simulink model "simpleThermalModel_v2"  (R2022a)
settings: Solver=VariableStepAuto  StartTime=0.0  StopTime=36000  RelTol=1e-3
libraries: fl_lib x161, nesl_utility x51
(part 1 of 2)
settings Model: Creator=BrunoMattos  LastModifiedBy=BrunoMattos
settings OptimizationCC: ZeroExternalMemoryAtStartup=off  ZeroInternalMemoryAtStartup=off
settings RTWCC: TargetLang=C++
settings GRTTargetCC: TargetLangStandard=C++11 (ISO)  CodeInterfacePackaging=C++ class

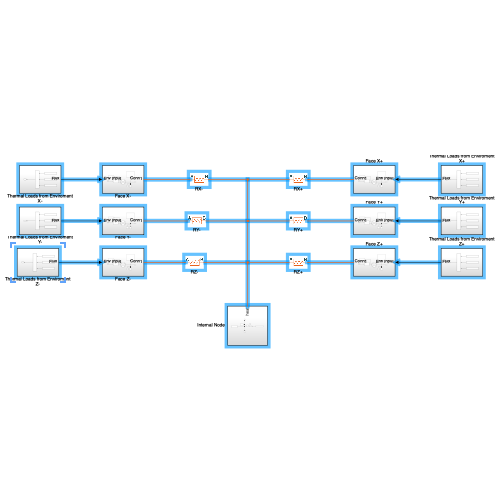
[thumbnail: Simulink's stored preview of the top-level diagram]
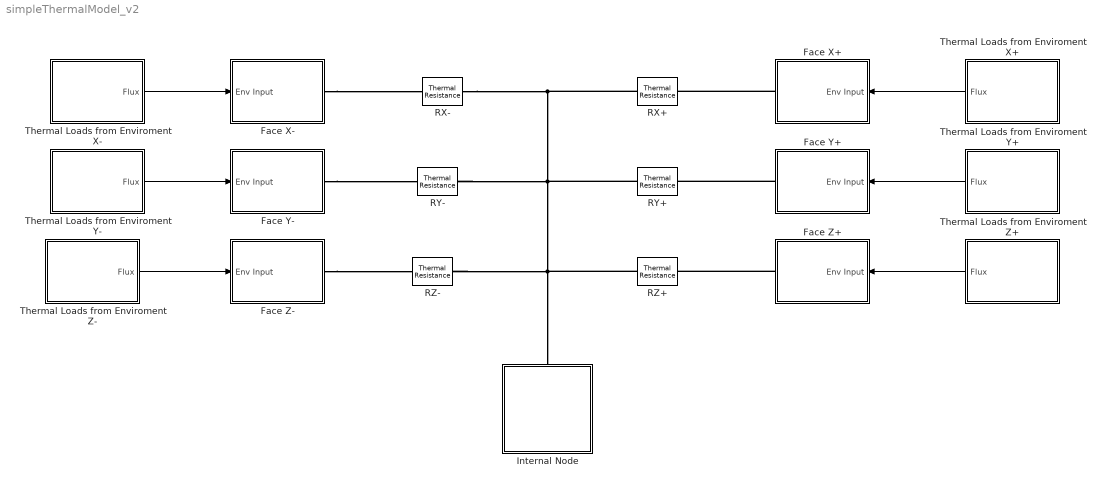
== system simpleThermalModel_v2 ==
  Face X+ : Subsystem
  Face X- : Subsystem
  Face Y+ : Subsystem
  Face Y- : Subsystem
  Face Z+ : Subsystem
  Face Z- : Subsystem
  Internal Node : Subsystem
  RX+ : fl_lib/Thermal/Thermal Elements/Thermal Resistance  resistance=0 K/W  T_specify=off  T_priority=None  T=0 K  T_nominal_specify=off  T_nominal_unit=K  T_nominal_value=1  Q_specify=off  Q_priority=None  Q=0 W  Q_nominal_specify=off  Q_nominal_unit=W  Q_nominal_value=1
      settings: SourceProductBaseCode=PW,SS,VE
  RX- : fl_lib/Thermal/Thermal Elements/Thermal Resistance  resistance=0 K/W  T_specify=off  T_priority=None  T=0 K  T_nominal_specify=off  T_nominal_unit=K  T_nominal_value=1  Q_specify=off  Q_priority=None  Q=0 W  Q_nominal_specify=off  Q_nominal_unit=W  Q_nominal_value=1
      settings: SourceProductBaseCode=PW,SS,VE
  RY+ : fl_lib/Thermal/Thermal Elements/Thermal Resistance  resistance=0 K/W  T_specify=off  T_priority=None  T=0 K  T_nominal_specify=off  T_nominal_unit=K  T_nominal_value=1  Q_specify=off  Q_priority=None  Q=0 W  Q_nominal_specify=off  Q_nominal_unit=W  Q_nominal_value=1
      settings: SourceProductBaseCode=PW,SS,VE
  RY- : fl_lib/Thermal/Thermal Elements/Thermal Resistance  resistance=0 K/W  T_specify=off  T_priority=None  T=0 K  T_nominal_specify=off  T_nominal_unit=K  T_nominal_value=1  Q_specify=off  Q_priority=None  Q=0 W  Q_nominal_specify=off  Q_nominal_unit=W  Q_nominal_value=1
      settings: SourceProductBaseCode=PW,SS,VE
  RZ+ : fl_lib/Thermal/Thermal Elements/Thermal Resistance  resistance=0 K/W  T_specify=off  T_priority=None  T=0 K  T_nominal_specify=off  T_nominal_unit=K  T_nominal_value=1  Q_specify=off  Q_priority=None  Q=0 W  Q_nominal_specify=off  Q_nominal_unit=W  Q_nominal_value=1
      settings: SourceProductBaseCode=PW,SS,VE
  RZ- : fl_lib/Thermal/Thermal Elements/Thermal Resistance  resistance=0 K/W  T_specify=off  T_priority=None  T=0 K  T_nominal_specify=off  T_nominal_unit=K  T_nominal_value=1  Q_specify=off  Q_priority=None  Q=0 W  Q_nominal_specify=off  Q_nominal_unit=W  Q_nominal_value=1
      settings: SourceProductBaseCode=PW,SS,VE
  Thermal Loads from Enviroment X+ : Subsystem
  Thermal Loads from Enviroment X- : Subsystem
  Thermal Loads from Enviroment Y+ : Subsystem
  Thermal Loads from Enviroment Y- : Subsystem
  Thermal Loads from Enviroment Z+ : Subsystem
  Thermal Loads from Enviroment Z- : Subsystem
  wires:
  Thermal Loads from Enviroment X+/1(Flux) -> Face X+/1(Env Input)
  Thermal Loads from Enviroment Y+/1(Flux) -> Face Y+/1(Env Input)
  Thermal Loads from Enviroment Z+/1(Flux) -> Face Z+/1(Env Input)
  Thermal Loads from Enviroment X-/1(Flux) -> Face X-/1(Env Input)
  Thermal Loads from Enviroment Y-/1(Flux) -> Face Y-/1(Env Input)
  Thermal Loads from Enviroment Z-/1(Flux) -> Face Z-/1(Env Input)
  connections:
  RX+/LConn1 -- RX-/RConn1 -- RZ-/RConn1 -- Internal Node/LConn1 -- RZ+/LConn1 -- RY-/RConn1 -- RY+/LConn1
  Face X-/RConn1 -- RX-/LConn1
  Face Y-/RConn1 -- RY-/LConn1
  Face Z-/RConn1 -- RZ-/LConn1
  Face X+/RConn1 -- RX+/RConn1
  Face Y+/RConn1 -- RY+/RConn1
  Face Z+/RConn1 -- RZ+/RConn1

== system simpleThermalModel_v2/Face X+ ==
  Env Input : Inport
  Inner Face Temp : Subsystem
  Neighboor Faces : Subsystem
  OuterLayer : Subsystem
  R_Blanket : fl_lib/Thermal/Thermal Elements/Thermal Resistance  resistance=0 K/W  T_specify=off  T_priority=None  T=0 K  T_nominal_specify=off  T_nominal_unit=K  T_nominal_value=1  Q_specify=off  Q_priority=None  Q=0 W  Q_nominal_specify=off  Q_nominal_unit=W  Q_nominal_value=1
      settings: SourceProductBaseCode=PW,SS,VE
  RadHeatBlanket : fl_lib/Thermal/Thermal Elements/Radiative Heat Transfer  area=1 m^2  rad_tr_coeff=1 W/(K^4*m^2)  T_specify=off  T_priority=None  T=0 K  T_nominal_specify=off  T_nominal_unit=K  T_nominal_value=1  Q_specify=off  Q_priority=None  Q=0 W  Q_nominal_specify=off  Q_nominal_unit=W  Q_nominal_value=1
      settings: SourceProductBaseCode=PW,SS,VE  InternalSimscapePortConfiguration="{\"Bottom\":[],\"Left\":[{\"id\":\"A\",\"label\":\"A\",\"type\":\"foundation.thermal.thermal\"}],\"Right\":[{\"id\":\"B\",\"label\":\"B\",\"type\":\"foundation.thermal.thermal\"}],\"Top\":[]}"
  Thermal Mass : fl_lib/Thermal/Thermal Elements/Thermal Mass  mass=1 kg  sp_heat=1 J/(K*kg)  T_specify=off  T_priority=High  T=300 K  T_nominal_specify=off  T_nominal_unit=K  T_nominal_value=1  Q_specify=off  Q_priority=None  Q=0 W  Q_nominal_specify=off  Q_nominal_unit=W  Q_nominal_value=1
      settings: SourceProductBaseCode=PW,SS,VE
  To Workspace : ToWorkspace  VariableName=XplusIRfluxOut  SaveFormat=Timeseries  SampleTime=-1
  Conn1 : PMIOPort  Side=Right
  wires:
  Env Input/1 -> OuterLayer/1(Env Input)
  OuterLayer/1(IR output) -> To Workspace/1
  connections:
  R_Blanket/RConn1 -- RadHeatBlanket/LConn1 -- Neighboor Faces/LConn1 -- Conn1/RConn1 -- Inner Face Temp/LConn1 -- Thermal Mass/LConn1
  OuterLayer/RConn1 -- RadHeatBlanket/RConn1 -- R_Blanket/LConn1

== system simpleThermalModel_v2/Face X- ==
  Env Input : Inport
  Inner Face Temp : Subsystem
  Neighboor Faces : Subsystem
  OuterLayer : Subsystem
  R_Blanket : fl_lib/Thermal/Thermal Elements/Thermal Resistance  resistance=0 K/W  T_specify=off  T_priority=None  T=0 K  T_nominal_specify=off  T_nominal_unit=K  T_nominal_value=1  Q_specify=off  Q_priority=None  Q=0 W  Q_nominal_specify=off  Q_nominal_unit=W  Q_nominal_value=1
      settings: SourceProductBaseCode=PW,SS,VE
  RadHeatBlanket : fl_lib/Thermal/Thermal Elements/Radiative Heat Transfer  area=1 m^2  rad_tr_coeff=1 W/(K^4*m^2)  T_specify=off  T_priority=None  T=0 K  T_nominal_specify=off  T_nominal_unit=K  T_nominal_value=1  Q_specify=off  Q_priority=None  Q=0 W  Q_nominal_specify=off  Q_nominal_unit=W  Q_nominal_value=1
      settings: SourceProductBaseCode=PW,SS,VE  InternalSimscapePortConfiguration="{\"Bottom\":[],\"Left\":[{\"id\":\"A\",\"label\":\"A\",\"type\":\"foundation.thermal.thermal\"}],\"Right\":[{\"id\":\"B\",\"label\":\"B\",\"type\":\"foundation.thermal.thermal\"}],\"Top\":[]}"
  Thermal Mass : fl_lib/Thermal/Thermal Elements/Thermal Mass  mass=1 kg  sp_heat=1 J/(K*kg)  T_specify=off  T_priority=High  T=300 K  T_nominal_specify=off  T_nominal_unit=K  T_nominal_value=1  Q_specify=off  Q_priority=None  Q=0 W  Q_nominal_specify=off  Q_nominal_unit=W  Q_nominal_value=1
      settings: SourceProductBaseCode=PW,SS,VE
  To Workspace : ToWorkspace  VariableName=XminusIRfluxOut  SaveFormat=Timeseries  SampleTime=-1
  Conn1 : PMIOPort  Side=Right
  wires:
  Env Input/1 -> OuterLayer/1(Env Input)
  OuterLayer/1(IR output) -> To Workspace/1
  connections:
  Neighboor Faces/LConn1 -- Conn1/RConn1 -- Inner Face Temp/LConn1 -- Thermal Mass/LConn1 -- R_Blanket/RConn1 -- RadHeatBlanket/LConn1
  OuterLayer/RConn1 -- R_Blanket/LConn1 -- RadHeatBlanket/RConn1

== system simpleThermalModel_v2/Face Y+ ==
  Env Input : Inport
  Inner Face Temp : Subsystem
  Neighboor Faces : Subsystem
  OuterLayer : Subsystem
  R_Blanket : fl_lib/Thermal/Thermal Elements/Thermal Resistance  resistance=0 K/W  T_specify=off  T_priority=None  T=0 K  T_nominal_specify=off  T_nominal_unit=K  T_nominal_value=1  Q_specify=off  Q_priority=None  Q=0 W  Q_nominal_specify=off  Q_nominal_unit=W  Q_nominal_value=1
      settings: SourceProductBaseCode=PW,SS,VE
  RadHeatBlanket : fl_lib/Thermal/Thermal Elements/Radiative Heat Transfer  area=1 m^2  rad_tr_coeff=1 W/(K^4*m^2)  T_specify=off  T_priority=None  T=0 K  T_nominal_specify=off  T_nominal_unit=K  T_nominal_value=1  Q_specify=off  Q_priority=None  Q=0 W  Q_nominal_specify=off  Q_nominal_unit=W  Q_nominal_value=1
      settings: SourceProductBaseCode=PW,SS,VE  InternalSimscapePortConfiguration="{\"Bottom\":[],\"Left\":[{\"id\":\"A\",\"label\":\"A\",\"type\":\"foundation.thermal.thermal\"}],\"Right\":[{\"id\":\"B\",\"label\":\"B\",\"type\":\"foundation.thermal.thermal\"}],\"Top\":[]}"
  Thermal Mass : fl_lib/Thermal/Thermal Elements/Thermal Mass  mass=1 kg  sp_heat=1 J/(K*kg)  T_specify=off  T_priority=High  T=300 K  T_nominal_specify=off  T_nominal_unit=K  T_nominal_value=1  Q_specify=off  Q_priority=None  Q=0 W  Q_nominal_specify=off  Q_nominal_unit=W  Q_nominal_value=1
      settings: SourceProductBaseCode=PW,SS,VE
  To Workspace : ToWorkspace  VariableName=YplusIRfluxOut  SaveFormat=Timeseries  SampleTime=-1
  Conn1 : PMIOPort  Side=Right
  wires:
  Env Input/1 -> OuterLayer/1(Env Input)
  OuterLayer/1(IR output) -> To Workspace/1
  connections:
  Neighboor Faces/LConn1 -- Conn1/RConn1 -- Inner Face Temp/LConn1 -- Thermal Mass/LConn1 -- R_Blanket/RConn1 -- RadHeatBlanket/LConn1
  OuterLayer/RConn1 -- R_Blanket/LConn1 -- RadHeatBlanket/RConn1

== system simpleThermalModel_v2/Face Y- ==
  Env Input : Inport
  Inner Face Temp : Subsystem
  Neighboor Faces : Subsystem
  OuterLayer : Subsystem
  R_Blanket : fl_lib/Thermal/Thermal Elements/Thermal Resistance  resistance=0 K/W  T_specify=off  T_priority=None  T=0 K  T_nominal_specify=off  T_nominal_unit=K  T_nominal_value=1  Q_specify=off  Q_priority=None  Q=0 W  Q_nominal_specify=off  Q_nominal_unit=W  Q_nominal_value=1
      settings: SourceProductBaseCode=PW,SS,VE
  RadHeatBlanket : fl_lib/Thermal/Thermal Elements/Radiative Heat Transfer  area=1 m^2  rad_tr_coeff=1 W/(K^4*m^2)  T_specify=off  T_priority=None  T=0 K  T_nominal_specify=off  T_nominal_unit=K  T_nominal_value=1  Q_specify=off  Q_priority=None  Q=0 W  Q_nominal_specify=off  Q_nominal_unit=W  Q_nominal_value=1
      settings: SourceProductBaseCode=PW,SS,VE  InternalSimscapePortConfiguration="{\"Bottom\":[],\"Left\":[{\"id\":\"A\",\"label\":\"A\",\"type\":\"foundation.thermal.thermal\"}],\"Right\":[{\"id\":\"B\",\"label\":\"B\",\"type\":\"foundation.thermal.thermal\"}],\"Top\":[]}"
  Thermal Mass : fl_lib/Thermal/Thermal Elements/Thermal Mass  mass=1 kg  sp_heat=1 J/(K*kg)  T_specify=off  T_priority=High  T=300 K  T_nominal_specify=off  T_nominal_unit=K  T_nominal_value=1  Q_specify=off  Q_priority=None  Q=0 W  Q_nominal_specify=off  Q_nominal_unit=W  Q_nominal_value=1
      settings: SourceProductBaseCode=PW,SS,VE
  To Workspace : ToWorkspace  VariableName=YminusIRfluxOut  SaveFormat=Timeseries  SampleTime=-1
  Conn1 : PMIOPort  Side=Right
  wires:
  Env Input/1 -> OuterLayer/1(Env Input)
  OuterLayer/1(IR output) -> To Workspace/1
  connections:
  Neighboor Faces/LConn1 -- Conn1/RConn1 -- Inner Face Temp/LConn1 -- Thermal Mass/LConn1 -- R_Blanket/RConn1 -- RadHeatBlanket/LConn1
  OuterLayer/RConn1 -- R_Blanket/LConn1 -- RadHeatBlanket/RConn1

== system simpleThermalModel_v2/Face Z+ ==
  Env Input : Inport
  Inner Face Temp : Subsystem
  Neighboor Faces : Subsystem
  OuterLayer : Subsystem
  R_Blanket : fl_lib/Thermal/Thermal Elements/Thermal Resistance  resistance=0 K/W  T_specify=off  T_priority=None  T=0 K  T_nominal_specify=off  T_nominal_unit=K  T_nominal_value=1  Q_specify=off  Q_priority=None  Q=0 W  Q_nominal_specify=off  Q_nominal_unit=W  Q_nominal_value=1
      settings: SourceProductBaseCode=PW,SS,VE
  RadHeatBlanket : fl_lib/Thermal/Thermal Elements/Radiative Heat Transfer  area=1 m^2  rad_tr_coeff=1 W/(K^4*m^2)  T_specify=off  T_priority=None  T=0 K  T_nominal_specify=off  T_nominal_unit=K  T_nominal_value=1  Q_specify=off  Q_priority=None  Q=0 W  Q_nominal_specify=off  Q_nominal_unit=W  Q_nominal_value=1
      settings: SourceProductBaseCode=PW,SS,VE  InternalSimscapePortConfiguration="{\"Bottom\":[],\"Left\":[{\"id\":\"A\",\"label\":\"A\",\"type\":\"foundation.thermal.thermal\"}],\"Right\":[{\"id\":\"B\",\"label\":\"B\",\"type\":\"foundation.thermal.thermal\"}],\"Top\":[]}"
  Thermal Mass : fl_lib/Thermal/Thermal Elements/Thermal Mass  mass=1 kg  sp_heat=1 J/(K*kg)  T_specify=off  T_priority=High  T=300 K  T_nominal_specify=off  T_nominal_unit=K  T_nominal_value=1  Q_specify=off  Q_priority=None  Q=0 W  Q_nominal_specify=off  Q_nominal_unit=W  Q_nominal_value=1
      settings: SourceProductBaseCode=PW,SS,VE
  To Workspace : ToWorkspace  VariableName=ZplusIRfluxOut  SaveFormat=Timeseries  SampleTime=-1
  Conn1 : PMIOPort  Side=Right
  wires:
  Env Input/1 -> OuterLayer/1(Env Input)
  OuterLayer/1(IR output) -> To Workspace/1
  connections:
  Neighboor Faces/LConn1 -- Conn1/RConn1 -- Inner Face Temp/LConn1 -- Thermal Mass/LConn1 -- R_Blanket/RConn1 -- RadHeatBlanket/LConn1
  OuterLayer/RConn1 -- R_Blanket/LConn1 -- RadHeatBlanket/RConn1

== system simpleThermalModel_v2/Face Z- ==
  Env Input : Inport
  Inner Face Temp : Subsystem
  Neighboor Faces : Subsystem
  OuterLayer : Subsystem
  R_Blanket : fl_lib/Thermal/Thermal Elements/Thermal Resistance  resistance=0 K/W  T_specify=off  T_priority=None  T=0 K  T_nominal_specify=off  T_nominal_unit=K  T_nominal_value=1  Q_specify=off  Q_priority=None  Q=0 W  Q_nominal_specify=off  Q_nominal_unit=W  Q_nominal_value=1
      settings: SourceProductBaseCode=PW,SS,VE
  RadHeatBlanket : fl_lib/Thermal/Thermal Elements/Radiative Heat Transfer  area=1 m^2  rad_tr_coeff=1 W/(K^4*m^2)  T_specify=off  T_priority=None  T=0 K  T_nominal_specify=off  T_nominal_unit=K  T_nominal_value=1  Q_specify=off  Q_priority=None  Q=0 W  Q_nominal_specify=off  Q_nominal_unit=W  Q_nominal_value=1
      settings: SourceProductBaseCode=PW,SS,VE  InternalSimscapePortConfiguration="{\"Bottom\":[],\"Left\":[{\"id\":\"A\",\"label\":\"A\",\"type\":\"foundation.thermal.thermal\"}],\"Right\":[{\"id\":\"B\",\"label\":\"B\",\"type\":\"foundation.thermal.thermal\"}],\"Top\":[]}"
  Thermal Mass : fl_lib/Thermal/Thermal Elements/Thermal Mass  mass=1 kg  sp_heat=1 J/(K*kg)  T_specify=off  T_priority=High  T=300 K  T_nominal_specify=off  T_nominal_unit=K  T_nominal_value=1  Q_specify=off  Q_priority=None  Q=0 W  Q_nominal_specify=off  Q_nominal_unit=W  Q_nominal_value=1
      settings: SourceProductBaseCode=PW,SS,VE
  To Workspace : ToWorkspace  VariableName=ZminusIRfluxOut  SaveFormat=Timeseries  SampleTime=-1
  Conn1 : PMIOPort  Side=Right
  wires:
  Env Input/1 -> OuterLayer/1(Env Input)
  OuterLayer/1(IR output) -> To Workspace/1
  connections:
  Neighboor Faces/LConn1 -- Conn1/RConn1 -- Inner Face Temp/LConn1 -- Thermal Mass/LConn1 -- R_Blanket/RConn1 -- RadHeatBlanket/LConn1
  OuterLayer/RConn1 -- R_Blanket/LConn1 -- RadHeatBlanket/RConn1

== system simpleThermalModel_v2/Internal Node ==
  Controlled Heat Flow Rate Source6 : fl_lib/Thermal/Thermal Sources/Controlled Heat Flow Rate Source
      settings: SourceProductBaseCode=PW,SS,VE
  Internal Node 1 : fl_lib/Thermal/Thermal Elements/Thermal Mass  mass=1 kg  sp_heat=1 J/(K*kg)  T_specify=off  T_priority=High  T=300 K  T_nominal_specify=off  T_nominal_unit=K  T_nominal_value=1  Q_specify=off  Q_priority=None  Q=0 W  Q_nominal_specify=off  Q_nominal_unit=W  Q_nominal_value=1
      settings: SourceProductBaseCode=PW,SS,VE
  Internal Node Pwr : FromWorkspace  VariableName=[0,0]
  Simulink-PS Converter6 : nesl_utility/Simulink-PS Converter  PhysicalDomain=network_engine_domain  SubClassName=ps_input  LeftPortType=input  RightPortType=output  PseudoPeriodic=off  Frequencies=[]  NoiseDistribution=none  NoiseParameters=[]  Unit=1  AffineConversion=off  FilteringAndDerivatives=provide  SimscapeFilterOrder=1  InputFilterTimeConstant=0.001  UdotUserProvided=0
      settings: SourceProductBaseCode=SS,PW,VE
  Solver Configuration : nesl_utility/Solver Configuration  PhysicalDomain=network_engine_domain  SubClassName=solver  LeftPortType=input  RightPortType=generic  Tones=[]  Harmonics=[]  SimulateNoise=off  Profile=off  UseLocalSampling=off  EnableSwitchedLinearOptims=on  FrequencyDomain=off  UseCCode=off  RelTol=0.001  AbsTol=0.001  MinStep=1e-09  ToWorkspace=off  RevertToSquareIcSolve=off  NumHomotopyIterations=100  PhasorMode=off  PhasorModeNumHarmonics=1  IndexReductionMethod=DerivativeReplacement  DoDC=off  ResidualTolerance=1e-09  UseLocalSolver=off  LocalSolverChoice=NE_BACKWARD_EULER_ADVANCER  LocalSolverSampleTime=0.001  DoFixedCost=off  MaxNonlinIter=3  MaxModeIter=2  ComputeImpulses=off  ImpulseIterations=2  LinearAlgebra=auto  LinearAlgebraNumThread=0  EquationFormulation=NE_TIME_EF  DelaysMemoryBudget=1024  AutomaticFiltering=on  FilteringTimeConstant=0.001  PartitionStorageMethod=AS_NEEDED  PartitionMemoryBudget=1024  PartitionMethod=ROBUST
      settings: SourceProductBaseCode=SS,PW,VE
  Temp Sensor : Subsystem
  Thermal Reference7 : fl_lib/Thermal/Thermal Elements/Thermal Reference
      settings: SourceProductBaseCode=PW,SS,VE
  heat : PMIOPort  Side=Left
  wires:
  Internal Node Pwr/1 -> Simulink-PS Converter6/1
  connections:
  Controlled Heat Flow Rate Source6/RConn1 -- Simulink-PS Converter6/RConn1
  Thermal Reference7/LConn1 -- Controlled Heat Flow Rate Source6/RConn2
  Temp Sensor/LConn1 -- heat/RConn1 -- Solver Configuration/RConn1 -- Controlled Heat Flow Rate Source6/LConn1 -- Internal Node 1/LConn1

== system simpleThermalModel_v2/Thermal Loads from Enviroment X+ ==
  Add : Sum  Inputs=+++
  Albedo Flux : FromWorkspace  VariableName=[0,0]
  IR Flux : FromWorkspace  VariableName=[0,0]
  Solar Flux : FromWorkspace  VariableName=[0,0]
  Flux : Outport
  wires:
  Albedo Flux/1 -> Add/3
  Solar Flux/1 -> Add/1
  Add/1 -> Flux/1
  IR Flux/1 -> Add/2

== system simpleThermalModel_v2/Thermal Loads from Enviroment X- ==
  Add : Sum  Inputs=+++
  Albedo Flux : FromWorkspace  VariableName=[0,0]
  IR Flux : FromWorkspace  VariableName=[0,0]
  Solar Flux : FromWorkspace  VariableName=[0,0]
  Flux : Outport
  wires:
  Albedo Flux/1 -> Add/3
  Solar Flux/1 -> Add/1
  Add/1 -> Flux/1
  IR Flux/1 -> Add/2

== system simpleThermalModel_v2/Thermal Loads from Enviroment Y+ ==
  Add : Sum  Inputs=+++
  Albedo Flux : FromWorkspace  VariableName=[0,0]
  IR Flux : FromWorkspace  VariableName=[0,0]
  Solar Flux : FromWorkspace  VariableName=[0,0]
  Flux : Outport
  wires:
  Albedo Flux/1 -> Add/3
  Solar Flux/1 -> Add/1
  Add/1 -> Flux/1
  IR Flux/1 -> Add/2

== system simpleThermalModel_v2/Thermal Loads from Enviroment Y- ==
  Add : Sum  Inputs=+++
  Albedo Flux : FromWorkspace  VariableName=[0,0]
  IR Flux : FromWorkspace  VariableName=[0,0]
  Solar Flux : FromWorkspace  VariableName=[0,0]
  Flux : Outport
  wires:
  Albedo Flux/1 -> Add/3
  Solar Flux/1 -> Add/1
  Add/1 -> Flux/1
  IR Flux/1 -> Add/2

== system simpleThermalModel_v2/Thermal Loads from Enviroment Z+ ==
  Add : Sum  Inputs=+++
  Albedo Flux : FromWorkspace  VariableName=[0,0]
  IR Flux : FromWorkspace  VariableName=[0,0]
  Solar Flux : FromWorkspace  VariableName=[0,0]
  Flux : Outport
  wires:
  Albedo Flux/1 -> Add/3
  Solar Flux/1 -> Add/1
  Add/1 -> Flux/1
  IR Flux/1 -> Add/2

== system simpleThermalModel_v2/Thermal Loads from Enviroment Z- ==
  Add : Sum  Inputs=+++
  Albedo Flux : FromWorkspace  VariableName=[0,0]
  IR Flux : FromWorkspace  VariableName=[0,0]
  Solar Flux : FromWorkspace  VariableName=[0,0]
  Flux : Outport
  wires:
  Albedo Flux/1 -> Add/3
  Solar Flux/1 -> Add/1
  Add/1 -> Flux/1
  IR Flux/1 -> Add/2

== system simpleThermalModel_v2/Face X+/Inner Face Temp ==
  PS-Simulink Converter : nesl_utility/PS-Simulink Converter  PhysicalDomain=network_engine_domain  SubClassName=ps_output  LeftPortType=input  RightPortType=output  PseudoPeriodic=off  Frequencies=[]  VectorFormat=inherit  Unit=inherit  AffineConversion=off
      settings: SourceProductBaseCode=SS,PW,VE
  Temperature Sensor : fl_lib/Thermal/Thermal Sensors/Temperature Sensor
      settings: SourceProductBaseCode=PW,SS,VE
  Thermal Reference1 : fl_lib/Thermal/Thermal Elements/Thermal Reference
      settings: SourceProductBaseCode=PW,SS,VE
  T_K : PMIOPort  Side=Left
  tag scope: InnerFaceTempXplus=global
  wires:
  PS-Simulink Converter/1 -> [InnerFaceTempXplus]
  connections:
  Temperature Sensor/LConn1 -- T_K/RConn1
  Temperature Sensor/RConn2 -- PS-Simulink Converter/LConn1
  Thermal Reference1/LConn1 -- Temperature Sensor/RConn1

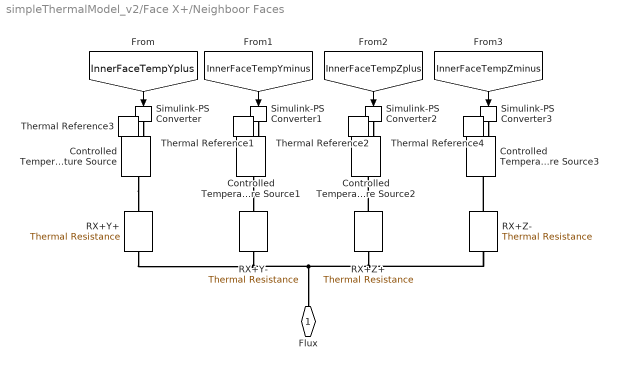
== system simpleThermalModel_v2/Face X+/Neighboor Faces ==
  Controlled Temperature Source{,1..3} (4 alike) : fl_lib/Thermal/Thermal Sources/Controlled Temperature Source
      settings: SourceProductBaseCode=PW,SS,VE
  RX+Y+ : fl_lib/Thermal/Thermal Elements/Thermal Resistance  resistance=0 K/W  T_specify=off  T_priority=None  T=0 K  T_nominal_specify=off  T_nominal_unit=K  T_nominal_value=1  Q_specify=off  Q_priority=None  Q=0 W  Q_nominal_specify=off  Q_nominal_unit=W  Q_nominal_value=1
      settings: SourceProductBaseCode=PW,SS,VE
  RX+Y- : fl_lib/Thermal/Thermal Elements/Thermal Resistance  resistance=0 K/W  T_specify=off  T_priority=None  T=0 K  T_nominal_specify=off  T_nominal_unit=K  T_nominal_value=1  Q_specify=off  Q_priority=None  Q=0 W  Q_nominal_specify=off  Q_nominal_unit=W  Q_nominal_value=1
      settings: SourceProductBaseCode=PW,SS,VE
  RX+Z+ : fl_lib/Thermal/Thermal Elements/Thermal Resistance  resistance=0 K/W  T_specify=off  T_priority=None  T=0 K  T_nominal_specify=off  T_nominal_unit=K  T_nominal_value=1  Q_specify=off  Q_priority=None  Q=0 W  Q_nominal_specify=off  Q_nominal_unit=W  Q_nominal_value=1
      settings: SourceProductBaseCode=PW,SS,VE
  RX+Z- : fl_lib/Thermal/Thermal Elements/Thermal Resistance  resistance=0 K/W  T_specify=off  T_priority=None  T=0 K  T_nominal_specify=off  T_nominal_unit=K  T_nominal_value=1  Q_specify=off  Q_priority=None  Q=0 W  Q_nominal_specify=off  Q_nominal_unit=W  Q_nominal_value=1
      settings: SourceProductBaseCode=PW,SS,VE
  Simulink-PS Converter{,1..3} (4 alike) : nesl_utility/Simulink-PS Converter  PhysicalDomain=network_engine_domain  SubClassName=ps_input  LeftPortType=input  RightPortType=output  PseudoPeriodic=off  Frequencies=[]  NoiseDistribution=none  NoiseParameters=[]  Unit=1  AffineConversion=off  FilteringAndDerivatives=provide  SimscapeFilterOrder=1  InputFilterTimeConstant=0.001  UdotUserProvided=0
      settings: SourceProductBaseCode=SS,PW,VE
  Thermal Reference{1..4} (4 alike) : fl_lib/Thermal/Thermal Elements/Thermal Reference
      settings: SourceProductBaseCode=PW,SS,VE
  Flux : PMIOPort  Side=Left
  wires:
  [InnerFaceTempYplus] -> Simulink-PS Converter/1
  [InnerFaceTempYminus] -> Simulink-PS Converter1/1
  [InnerFaceTempZplus] -> Simulink-PS Converter2/1
  [InnerFaceTempZminus] -> Simulink-PS Converter3/1
  connections:
  RX+Z-/RConn1 -- RX+Z+/RConn1 -- RX+Y+/RConn1 -- RX+Y-/RConn1 -- Flux/RConn1
  Simulink-PS Converter/RConn1 -- Controlled Temperature Source/RConn1
  Controlled Temperature Source/LConn1 -- RX+Y+/LConn1
  Thermal Reference3/LConn1 -- Controlled Temperature Source/RConn2
  Simulink-PS Converter1/RConn1 -- Controlled Temperature Source1/RConn1
  Thermal Reference1/LConn1 -- Controlled Temperature Source1/RConn2
  Controlled Temperature Source1/LConn1 -- RX+Y-/LConn1
  RX+Z+/LConn1 -- Controlled Temperature Source2/LConn1
  Thermal Reference2/LConn1 -- Controlled Temperature Source2/RConn2
  Simulink-PS Converter2/RConn1 -- Controlled Temperature Source2/RConn1
  RX+Z-/LConn1 -- Controlled Temperature Source3/LConn1
  Thermal Reference4/LConn1 -- Controlled Temperature Source3/RConn2
  Simulink-PS Converter3/RConn1 -- Controlled Temperature Source3/RConn1

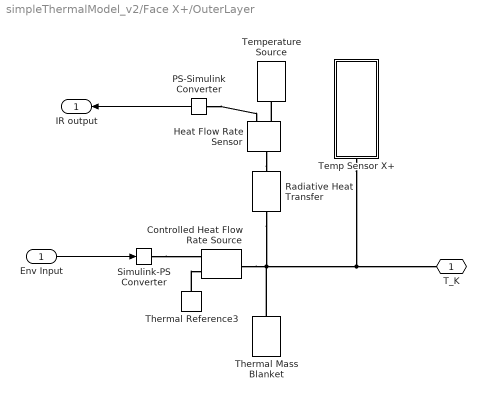
== system simpleThermalModel_v2/Face X+/OuterLayer ==
  Env Input : Inport
  Controlled Heat Flow Rate Source : fl_lib/Thermal/Thermal Sources/Controlled Heat Flow Rate Source
      settings: SourceProductBaseCode=PW,SS,VE
  Heat Flow Rate Sensor : fl_lib/Thermal/Thermal Sensors/Heat Flow Rate Sensor
      settings: SourceProductBaseCode=PW,SS,VE
  PS-Simulink Converter : nesl_utility/PS-Simulink Converter  PhysicalDomain=network_engine_domain  SubClassName=ps_output  LeftPortType=input  RightPortType=output  PseudoPeriodic=off  Frequencies=[]  VectorFormat=inherit  Unit=inherit  AffineConversion=off
      settings: SourceProductBaseCode=SS,PW,VE
  Radiative Heat Transfer : fl_lib/Thermal/Thermal Elements/Radiative Heat Transfer  area=1 m^2  rad_tr_coeff=1 W/(K^4*m^2)  T_specify=off  T_priority=None  T=0 K  T_nominal_specify=off  T_nominal_unit=K  T_nominal_value=1  Q_specify=off  Q_priority=None  Q=0 W  Q_nominal_specify=off  Q_nominal_unit=W  Q_nominal_value=1
      settings: SourceProductBaseCode=PW,SS,VE  InternalSimscapePortConfiguration="{\"Bottom\":[],\"Left\":[{\"id\":\"A\",\"label\":\"A\",\"type\":\"foundation.thermal.thermal\"}],\"Right\":[{\"id\":\"B\",\"label\":\"B\",\"type\":\"foundation.thermal.thermal\"}],\"Top\":[]}"
  Simulink-PS Converter : nesl_utility/Simulink-PS Converter  PhysicalDomain=network_engine_domain  SubClassName=ps_input  LeftPortType=input  RightPortType=output  PseudoPeriodic=off  Frequencies=[]  NoiseDistribution=none  NoiseParameters=[]  Unit=1  AffineConversion=off  FilteringAndDerivatives=provide  SimscapeFilterOrder=1  InputFilterTimeConstant=0.001  UdotUserProvided=0
      settings: SourceProductBaseCode=SS,PW,VE
  Temp Sensor X+ : Subsystem
  Temperature Source : fl_lib/Thermal/Thermal Sources/Temperature Source  temperature=7 K
      settings: SourceProductBaseCode=PW,SS,VE
  Thermal Mass Blanket : fl_lib/Thermal/Thermal Elements/Thermal Mass  mass=1 kg  sp_heat=1 J/(K*kg)  T_specify=off  T_priority=High  T=300 K  T_nominal_specify=off  T_nominal_unit=K  T_nominal_value=1  Q_specify=off  Q_priority=None  Q=0 W  Q_nominal_specify=off  Q_nominal_unit=W  Q_nominal_value=1
      settings: SourceProductBaseCode=PW,SS,VE
  Thermal Reference3 : fl_lib/Thermal/Thermal Elements/Thermal Reference
      settings: SourceProductBaseCode=PW,SS,VE
  T_K : PMIOPort  Side=Right
  IR output : Outport
  wires:
  Env Input/1 -> Simulink-PS Converter/1
  PS-Simulink Converter/1 -> IR output/1
  connections:
  Radiative Heat Transfer/LConn1 -- Controlled Heat Flow Rate Source/LConn1 -- Thermal Mass Blanket/LConn1 -- T_K/RConn1 -- Temp Sensor X+/LConn1
  Simulink-PS Converter/RConn1 -- Controlled Heat Flow Rate Source/RConn1
  Heat Flow Rate Sensor/LConn1 -- Radiative Heat Transfer/RConn1
  Heat Flow Rate Sensor/RConn2 -- Temperature Source/LConn1
  Thermal Reference3/LConn1 -- Controlled Heat Flow Rate Source/RConn2
  PS-Simulink Converter/LConn1 -- Heat Flow Rate Sensor/RConn1

== system simpleThermalModel_v2/Face X-/Inner Face Temp ==
  PS-Simulink Converter : nesl_utility/PS-Simulink Converter  PhysicalDomain=network_engine_domain  SubClassName=ps_output  LeftPortType=input  RightPortType=output  PseudoPeriodic=off  Frequencies=[]  VectorFormat=inherit  Unit=inherit  AffineConversion=off
      settings: SourceProductBaseCode=SS,PW,VE
  Temperature Sensor : fl_lib/Thermal/Thermal Sensors/Temperature Sensor
      settings: SourceProductBaseCode=PW,SS,VE
  Thermal Reference1 : fl_lib/Thermal/Thermal Elements/Thermal Reference
      settings: SourceProductBaseCode=PW,SS,VE
  T_K : PMIOPort  Side=Left
  tag scope: InnerFaceTempXminus=global
  wires:
  PS-Simulink Converter/1 -> [InnerFaceTempXminus]
  connections:
  Temperature Sensor/LConn1 -- T_K/RConn1
  Temperature Sensor/RConn2 -- PS-Simulink Converter/LConn1
  Thermal Reference1/LConn1 -- Temperature Sensor/RConn1

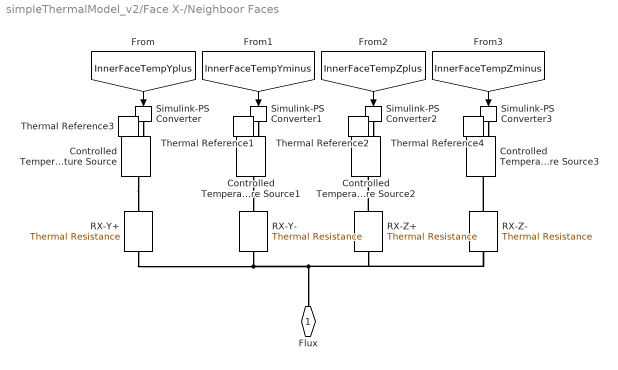
== system simpleThermalModel_v2/Face X-/Neighboor Faces ==
  Controlled Temperature Source{,1..3} (4 alike) : fl_lib/Thermal/Thermal Sources/Controlled Temperature Source
      settings: SourceProductBaseCode=PW,SS,VE
  RX-Y+ : fl_lib/Thermal/Thermal Elements/Thermal Resistance  resistance=0 K/W  T_specify=off  T_priority=None  T=0 K  T_nominal_specify=off  T_nominal_unit=K  T_nominal_value=1  Q_specify=off  Q_priority=None  Q=0 W  Q_nominal_specify=off  Q_nominal_unit=W  Q_nominal_value=1
      settings: SourceProductBaseCode=PW,SS,VE
  RX-Y- : fl_lib/Thermal/Thermal Elements/Thermal Resistance  resistance=0 K/W  T_specify=off  T_priority=None  T=0 K  T_nominal_specify=off  T_nominal_unit=K  T_nominal_value=1  Q_specify=off  Q_priority=None  Q=0 W  Q_nominal_specify=off  Q_nominal_unit=W  Q_nominal_value=1
      settings: SourceProductBaseCode=PW,SS,VE
  RX-Z+ : fl_lib/Thermal/Thermal Elements/Thermal Resistance  resistance=0 K/W  T_specify=off  T_priority=None  T=0 K  T_nominal_specify=off  T_nominal_unit=K  T_nominal_value=1  Q_specify=off  Q_priority=None  Q=0 W  Q_nominal_specify=off  Q_nominal_unit=W  Q_nominal_value=1
      settings: SourceProductBaseCode=PW,SS,VE
  RX-Z- : fl_lib/Thermal/Thermal Elements/Thermal Resistance  resistance=0 K/W  T_specify=off  T_priority=None  T=0 K  T_nominal_specify=off  T_nominal_unit=K  T_nominal_value=1  Q_specify=off  Q_priority=None  Q=0 W  Q_nominal_specify=off  Q_nominal_unit=W  Q_nominal_value=1
      settings: SourceProductBaseCode=PW,SS,VE
  Simulink-PS Converter{,1..3} (4 alike) : nesl_utility/Simulink-PS Converter  PhysicalDomain=network_engine_domain  SubClassName=ps_input  LeftPortType=input  RightPortType=output  PseudoPeriodic=off  Frequencies=[]  NoiseDistribution=none  NoiseParameters=[]  Unit=1  AffineConversion=off  FilteringAndDerivatives=provide  SimscapeFilterOrder=1  InputFilterTimeConstant=0.001  UdotUserProvided=0
      settings: SourceProductBaseCode=SS,PW,VE
  Thermal Reference{1..4} (4 alike) : fl_lib/Thermal/Thermal Elements/Thermal Reference
      settings: SourceProductBaseCode=PW,SS,VE
  Flux : PMIOPort  Side=Left
  wires:
  [InnerFaceTempYplus] -> Simulink-PS Converter/1
  [InnerFaceTempYminus] -> Simulink-PS Converter1/1
  [InnerFaceTempZplus] -> Simulink-PS Converter2/1
  [InnerFaceTempZminus] -> Simulink-PS Converter3/1
  connections:
  RX-Y+/RConn1 -- RX-Y-/RConn1 -- RX-Z-/RConn1 -- RX-Z+/RConn1 -- Flux/RConn1
  Simulink-PS Converter/RConn1 -- Controlled Temperature Source/RConn1
  Controlled Temperature Source/LConn1 -- RX-Y+/LConn1
  Thermal Reference3/LConn1 -- Controlled Temperature Source/RConn2
  Simulink-PS Converter1/RConn1 -- Controlled Temperature Source1/RConn1
  Thermal Reference1/LConn1 -- Controlled Temperature Source1/RConn2
  Controlled Temperature Source1/LConn1 -- RX-Y-/LConn1
  RX-Z+/LConn1 -- Controlled Temperature Source2/LConn1
  Thermal Reference2/LConn1 -- Controlled Temperature Source2/RConn2
  Simulink-PS Converter2/RConn1 -- Controlled Temperature Source2/RConn1
  RX-Z-/LConn1 -- Controlled Temperature Source3/LConn1
  Thermal Reference4/LConn1 -- Controlled Temperature Source3/RConn2
  Simulink-PS Converter3/RConn1 -- Controlled Temperature Source3/RConn1

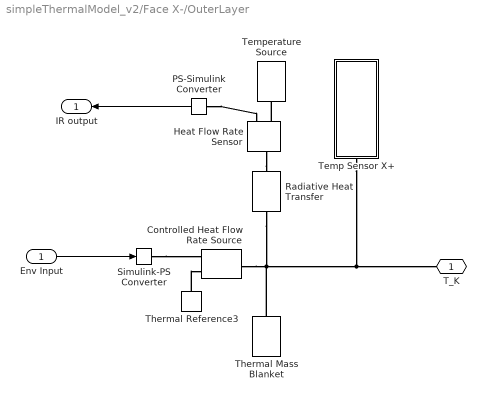
== system simpleThermalModel_v2/Face X-/OuterLayer ==
  Env Input : Inport
  Controlled Heat Flow Rate Source : fl_lib/Thermal/Thermal Sources/Controlled Heat Flow Rate Source
      settings: SourceProductBaseCode=PW,SS,VE
  Heat Flow Rate Sensor : fl_lib/Thermal/Thermal Sensors/Heat Flow Rate Sensor
      settings: SourceProductBaseCode=PW,SS,VE
  PS-Simulink Converter : nesl_utility/PS-Simulink Converter  PhysicalDomain=network_engine_domain  SubClassName=ps_output  LeftPortType=input  RightPortType=output  PseudoPeriodic=off  Frequencies=[]  VectorFormat=inherit  Unit=inherit  AffineConversion=off
      settings: SourceProductBaseCode=SS,PW,VE
  Radiative Heat Transfer : fl_lib/Thermal/Thermal Elements/Radiative Heat Transfer  area=1 m^2  rad_tr_coeff=1 W/(K^4*m^2)  T_specify=off  T_priority=None  T=0 K  T_nominal_specify=off  T_nominal_unit=K  T_nominal_value=1  Q_specify=off  Q_priority=None  Q=0 W  Q_nominal_specify=off  Q_nominal_unit=W  Q_nominal_value=1
      settings: SourceProductBaseCode=PW,SS,VE  InternalSimscapePortConfiguration="{\"Bottom\":[],\"Left\":[{\"id\":\"A\",\"label\":\"A\",\"type\":\"foundation.thermal.thermal\"}],\"Right\":[{\"id\":\"B\",\"label\":\"B\",\"type\":\"foundation.thermal.thermal\"}],\"Top\":[]}"
  Simulink-PS Converter : nesl_utility/Simulink-PS Converter  PhysicalDomain=network_engine_domain  SubClassName=ps_input  LeftPortType=input  RightPortType=output  PseudoPeriodic=off  Frequencies=[]  NoiseDistribution=none  NoiseParameters=[]  Unit=1  AffineConversion=off  FilteringAndDerivatives=provide  SimscapeFilterOrder=1  InputFilterTimeConstant=0.001  UdotUserProvided=0
      settings: SourceProductBaseCode=SS,PW,VE
  Temp Sensor X+ : Subsystem
  Temperature Source : fl_lib/Thermal/Thermal Sources/Temperature Source  temperature=7 K
      settings: SourceProductBaseCode=PW,SS,VE
  Thermal Mass Blanket : fl_lib/Thermal/Thermal Elements/Thermal Mass  mass=1 kg  sp_heat=1 J/(K*kg)  T_specify=off  T_priority=High  T=300 K  T_nominal_specify=off  T_nominal_unit=K  T_nominal_value=1  Q_specify=off  Q_priority=None  Q=0 W  Q_nominal_specify=off  Q_nominal_unit=W  Q_nominal_value=1
      settings: SourceProductBaseCode=PW,SS,VE
  Thermal Reference3 : fl_lib/Thermal/Thermal Elements/Thermal Reference
      settings: SourceProductBaseCode=PW,SS,VE
  T_K : PMIOPort  Side=Right
  IR output : Outport
  wires:
  Env Input/1 -> Simulink-PS Converter/1
  PS-Simulink Converter/1 -> IR output/1
  connections:
  Controlled Heat Flow Rate Source/LConn1 -- Thermal Mass Blanket/LConn1 -- Radiative Heat Transfer/LConn1 -- Temp Sensor X+/LConn1 -- T_K/RConn1
  Simulink-PS Converter/RConn1 -- Controlled Heat Flow Rate Source/RConn1
  Heat Flow Rate Sensor/LConn1 -- Radiative Heat Transfer/RConn1
  Heat Flow Rate Sensor/RConn2 -- Temperature Source/LConn1
  Thermal Reference3/LConn1 -- Controlled Heat Flow Rate Source/RConn2
  PS-Simulink Converter/LConn1 -- Heat Flow Rate Sensor/RConn1

== system simpleThermalModel_v2/Face Y+/Inner Face Temp ==
  PS-Simulink Converter : nesl_utility/PS-Simulink Converter  PhysicalDomain=network_engine_domain  SubClassName=ps_output  LeftPortType=input  RightPortType=output  PseudoPeriodic=off  Frequencies=[]  VectorFormat=inherit  Unit=inherit  AffineConversion=off
      settings: SourceProductBaseCode=SS,PW,VE
  Temperature Sensor : fl_lib/Thermal/Thermal Sensors/Temperature Sensor
      settings: SourceProductBaseCode=PW,SS,VE
  Thermal Reference1 : fl_lib/Thermal/Thermal Elements/Thermal Reference
      settings: SourceProductBaseCode=PW,SS,VE
  T_K : PMIOPort  Side=Left
  tag scope: InnerFaceTempYplus=global
  wires:
  PS-Simulink Converter/1 -> [InnerFaceTempYplus]
  connections:
  Temperature Sensor/LConn1 -- T_K/RConn1
  Temperature Sensor/RConn2 -- PS-Simulink Converter/LConn1
  Thermal Reference1/LConn1 -- Temperature Sensor/RConn1

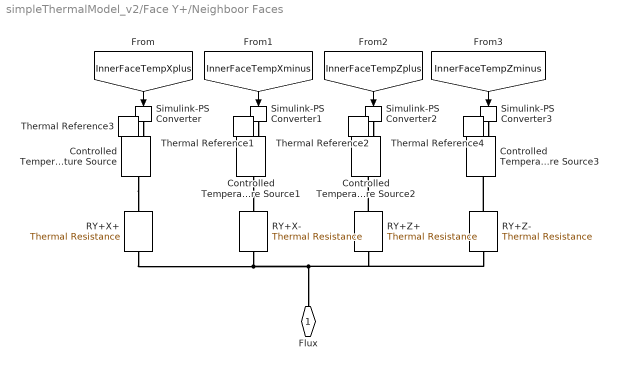
== system simpleThermalModel_v2/Face Y+/Neighboor Faces ==
  Controlled Temperature Source{,1..3} (4 alike) : fl_lib/Thermal/Thermal Sources/Controlled Temperature Source
      settings: SourceProductBaseCode=PW,SS,VE
  RY+X+ : fl_lib/Thermal/Thermal Elements/Thermal Resistance  resistance=0 K/W  T_specify=off  T_priority=None  T=0 K  T_nominal_specify=off  T_nominal_unit=K  T_nominal_value=1  Q_specify=off  Q_priority=None  Q=0 W  Q_nominal_specify=off  Q_nominal_unit=W  Q_nominal_value=1
      settings: SourceProductBaseCode=PW,SS,VE
  RY+X- : fl_lib/Thermal/Thermal Elements/Thermal Resistance  resistance=0 K/W  T_specify=off  T_priority=None  T=0 K  T_nominal_specify=off  T_nominal_unit=K  T_nominal_value=1  Q_specify=off  Q_priority=None  Q=0 W  Q_nominal_specify=off  Q_nominal_unit=W  Q_nominal_value=1
      settings: SourceProductBaseCode=PW,SS,VE
  RY+Z+ : fl_lib/Thermal/Thermal Elements/Thermal Resistance  resistance=0 K/W  T_specify=off  T_priority=None  T=0 K  T_nominal_specify=off  T_nominal_unit=K  T_nominal_value=1  Q_specify=off  Q_priority=None  Q=0 W  Q_nominal_specify=off  Q_nominal_unit=W  Q_nominal_value=1
      settings: SourceProductBaseCode=PW,SS,VE
  RY+Z- : fl_lib/Thermal/Thermal Elements/Thermal Resistance  resistance=0 K/W  T_specify=off  T_priority=None  T=0 K  T_nominal_specify=off  T_nominal_unit=K  T_nominal_value=1  Q_specify=off  Q_priority=None  Q=0 W  Q_nominal_specify=off  Q_nominal_unit=W  Q_nominal_value=1
      settings: SourceProductBaseCode=PW,SS,VE
  Simulink-PS Converter{,1..3} (4 alike) : nesl_utility/Simulink-PS Converter  PhysicalDomain=network_engine_domain  SubClassName=ps_input  LeftPortType=input  RightPortType=output  PseudoPeriodic=off  Frequencies=[]  NoiseDistribution=none  NoiseParameters=[]  Unit=1  AffineConversion=off  FilteringAndDerivatives=provide  SimscapeFilterOrder=1  InputFilterTimeConstant=0.001  UdotUserProvided=0
      settings: SourceProductBaseCode=SS,PW,VE
  Thermal Reference{1..4} (4 alike) : fl_lib/Thermal/Thermal Elements/Thermal Reference
      settings: SourceProductBaseCode=PW,SS,VE
  Flux : PMIOPort  Side=Left
  wires:
  [InnerFaceTempXplus] -> Simulink-PS Converter/1
  [InnerFaceTempXminus] -> Simulink-PS Converter1/1
  [InnerFaceTempZplus] -> Simulink-PS Converter2/1
  [InnerFaceTempZminus] -> Simulink-PS Converter3/1
  connections:
  RY+X+/RConn1 -- RY+X-/RConn1 -- RY+Z-/RConn1 -- RY+Z+/RConn1 -- Flux/RConn1
  Simulink-PS Converter/RConn1 -- Controlled Temperature Source/RConn1
  Controlled Temperature Source/LConn1 -- RY+X+/LConn1
  Thermal Reference3/LConn1 -- Controlled Temperature Source/RConn2
  Simulink-PS Converter1/RConn1 -- Controlled Temperature Source1/RConn1
  Thermal Reference1/LConn1 -- Controlled Temperature Source1/RConn2
  Controlled Temperature Source1/LConn1 -- RY+X-/LConn1
  RY+Z+/LConn1 -- Controlled Temperature Source2/LConn1
  Thermal Reference2/LConn1 -- Controlled Temperature Source2/RConn2
  Simulink-PS Converter2/RConn1 -- Controlled Temperature Source2/RConn1
  RY+Z-/LConn1 -- Controlled Temperature Source3/LConn1
  Thermal Reference4/LConn1 -- Controlled Temperature Source3/RConn2
  Simulink-PS Converter3/RConn1 -- Controlled Temperature Source3/RConn1

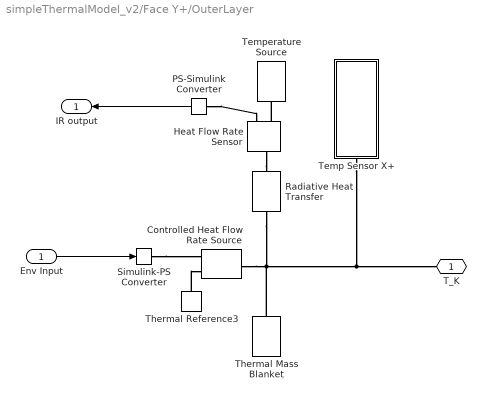
== system simpleThermalModel_v2/Face Y+/OuterLayer ==
  Env Input : Inport
  Controlled Heat Flow Rate Source : fl_lib/Thermal/Thermal Sources/Controlled Heat Flow Rate Source
      settings: SourceProductBaseCode=PW,SS,VE
  Heat Flow Rate Sensor : fl_lib/Thermal/Thermal Sensors/Heat Flow Rate Sensor
      settings: SourceProductBaseCode=PW,SS,VE
  PS-Simulink Converter : nesl_utility/PS-Simulink Converter  PhysicalDomain=network_engine_domain  SubClassName=ps_output  LeftPortType=input  RightPortType=output  PseudoPeriodic=off  Frequencies=[]  VectorFormat=inherit  Unit=inherit  AffineConversion=off
      settings: SourceProductBaseCode=SS,PW,VE
  Radiative Heat Transfer : fl_lib/Thermal/Thermal Elements/Radiative Heat Transfer  area=1 m^2  rad_tr_coeff=1 W/(K^4*m^2)  T_specify=off  T_priority=None  T=0 K  T_nominal_specify=off  T_nominal_unit=K  T_nominal_value=1  Q_specify=off  Q_priority=None  Q=0 W  Q_nominal_specify=off  Q_nominal_unit=W  Q_nominal_value=1
      settings: SourceProductBaseCode=PW,SS,VE  InternalSimscapePortConfiguration="{\"Bottom\":[],\"Left\":[{\"id\":\"A\",\"label\":\"A\",\"type\":\"foundation.thermal.thermal\"}],\"Right\":[{\"id\":\"B\",\"label\":\"B\",\"type\":\"foundation.thermal.thermal\"}],\"Top\":[]}"
  Simulink-PS Converter : nesl_utility/Simulink-PS Converter  PhysicalDomain=network_engine_domain  SubClassName=ps_input  LeftPortType=input  RightPortType=output  PseudoPeriodic=off  Frequencies=[]  NoiseDistribution=none  NoiseParameters=[]  Unit=1  AffineConversion=off  FilteringAndDerivatives=provide  SimscapeFilterOrder=1  InputFilterTimeConstant=0.001  UdotUserProvided=0
      settings: SourceProductBaseCode=SS,PW,VE
  Temp Sensor X+ : Subsystem
  Temperature Source : fl_lib/Thermal/Thermal Sources/Temperature Source  temperature=7 K
      settings: SourceProductBaseCode=PW,SS,VE
  Thermal Mass Blanket : fl_lib/Thermal/Thermal Elements/Thermal Mass  mass=1 kg  sp_heat=1 J/(K*kg)  T_specify=off  T_priority=High  T=300 K  T_nominal_specify=off  T_nominal_unit=K  T_nominal_value=1  Q_specify=off  Q_priority=None  Q=0 W  Q_nominal_specify=off  Q_nominal_unit=W  Q_nominal_value=1
      settings: SourceProductBaseCode=PW,SS,VE
  Thermal Reference3 : fl_lib/Thermal/Thermal Elements/Thermal Reference
      settings: SourceProductBaseCode=PW,SS,VE
  T_K : PMIOPort  Side=Right
  IR output : Outport
  wires:
  Env Input/1 -> Simulink-PS Converter/1
  PS-Simulink Converter/1 -> IR output/1
  connections:
  Controlled Heat Flow Rate Source/LConn1 -- Thermal Mass Blanket/LConn1 -- Radiative Heat Transfer/LConn1 -- Temp Sensor X+/LConn1 -- T_K/RConn1
  Simulink-PS Converter/RConn1 -- Controlled Heat Flow Rate Source/RConn1
  Heat Flow Rate Sensor/LConn1 -- Radiative Heat Transfer/RConn1
  Heat Flow Rate Sensor/RConn2 -- Temperature Source/LConn1
  Thermal Reference3/LConn1 -- Controlled Heat Flow Rate Source/RConn2
  PS-Simulink Converter/LConn1 -- Heat Flow Rate Sensor/RConn1

== system simpleThermalModel_v2/Face Y-/Inner Face Temp ==
  PS-Simulink Converter : nesl_utility/PS-Simulink Converter  PhysicalDomain=network_engine_domain  SubClassName=ps_output  LeftPortType=input  RightPortType=output  PseudoPeriodic=off  Frequencies=[]  VectorFormat=inherit  Unit=inherit  AffineConversion=off
      settings: SourceProductBaseCode=SS,PW,VE
  Temperature Sensor : fl_lib/Thermal/Thermal Sensors/Temperature Sensor
      settings: SourceProductBaseCode=PW,SS,VE
  Thermal Reference1 : fl_lib/Thermal/Thermal Elements/Thermal Reference
      settings: SourceProductBaseCode=PW,SS,VE
  T_K : PMIOPort  Side=Left
  tag scope: InnerFaceTempYminus=global
  wires:
  PS-Simulink Converter/1 -> [InnerFaceTempYminus]
  connections:
  Temperature Sensor/LConn1 -- T_K/RConn1
  Temperature Sensor/RConn2 -- PS-Simulink Converter/LConn1
  Thermal Reference1/LConn1 -- Temperature Sensor/RConn1

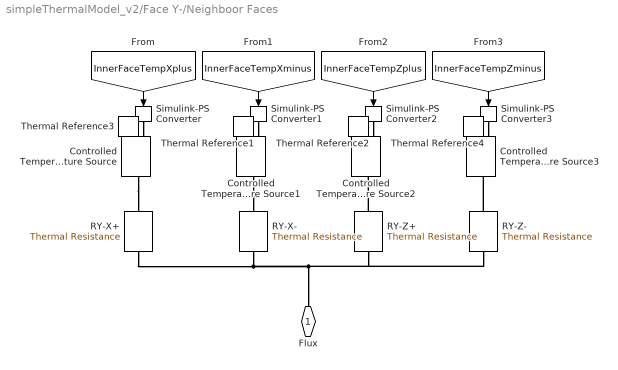
== system simpleThermalModel_v2/Face Y-/Neighboor Faces ==
  Controlled Temperature Source{,1..3} (4 alike) : fl_lib/Thermal/Thermal Sources/Controlled Temperature Source
      settings: SourceProductBaseCode=PW,SS,VE
  RY-X+ : fl_lib/Thermal/Thermal Elements/Thermal Resistance  resistance=0 K/W  T_specify=off  T_priority=None  T=0 K  T_nominal_specify=off  T_nominal_unit=K  T_nominal_value=1  Q_specify=off  Q_priority=None  Q=0 W  Q_nominal_specify=off  Q_nominal_unit=W  Q_nominal_value=1
      settings: SourceProductBaseCode=PW,SS,VE
  RY-X- : fl_lib/Thermal/Thermal Elements/Thermal Resistance  resistance=0 K/W  T_specify=off  T_priority=None  T=0 K  T_nominal_specify=off  T_nominal_unit=K  T_nominal_value=1  Q_specify=off  Q_priority=None  Q=0 W  Q_nominal_specify=off  Q_nominal_unit=W  Q_nominal_value=1
      settings: SourceProductBaseCode=PW,SS,VE
  RY-Z+ : fl_lib/Thermal/Thermal Elements/Thermal Resistance  resistance=0 K/W  T_specify=off  T_priority=None  T=0 K  T_nominal_specify=off  T_nominal_unit=K  T_nominal_value=1  Q_specify=off  Q_priority=None  Q=0 W  Q_nominal_specify=off  Q_nominal_unit=W  Q_nominal_value=1
      settings: SourceProductBaseCode=PW,SS,VE
  RY-Z- : fl_lib/Thermal/Thermal Elements/Thermal Resistance  resistance=0 K/W  T_specify=off  T_priority=None  T=0 K  T_nominal_specify=off  T_nominal_unit=K  T_nominal_value=1  Q_specify=off  Q_priority=None  Q=0 W  Q_nominal_specify=off  Q_nominal_unit=W  Q_nominal_value=1
      settings: SourceProductBaseCode=PW,SS,VE
  Simulink-PS Converter{,1..3} (4 alike) : nesl_utility/Simulink-PS Converter  PhysicalDomain=network_engine_domain  SubClassName=ps_input  LeftPortType=input  RightPortType=output  PseudoPeriodic=off  Frequencies=[]  NoiseDistribution=none  NoiseParameters=[]  Unit=1  AffineConversion=off  FilteringAndDerivatives=provide  SimscapeFilterOrder=1  InputFilterTimeConstant=0.001  UdotUserProvided=0
      settings: SourceProductBaseCode=SS,PW,VE
  Thermal Reference{1..4} (4 alike) : fl_lib/Thermal/Thermal Elements/Thermal Reference
      settings: SourceProductBaseCode=PW,SS,VE
  Flux : PMIOPort  Side=Left
  wires:
  [InnerFaceTempXplus] -> Simulink-PS Converter/1
  [InnerFaceTempXminus] -> Simulink-PS Converter1/1
  [InnerFaceTempZplus] -> Simulink-PS Converter2/1
  [InnerFaceTempZminus] -> Simulink-PS Converter3/1
  connections:
  RY-X+/RConn1 -- RY-X-/RConn1 -- RY-Z-/RConn1 -- RY-Z+/RConn1 -- Flux/RConn1
  Simulink-PS Converter/RConn1 -- Controlled Temperature Source/RConn1
  Controlled Temperature Source/LConn1 -- RY-X+/LConn1
  Thermal Reference3/LConn1 -- Controlled Temperature Source/RConn2
  Simulink-PS Converter1/RConn1 -- Controlled Temperature Source1/RConn1
  Thermal Reference1/LConn1 -- Controlled Temperature Source1/RConn2
  Controlled Temperature Source1/LConn1 -- RY-X-/LConn1
  RY-Z+/LConn1 -- Controlled Temperature Source2/LConn1
  Thermal Reference2/LConn1 -- Controlled Temperature Source2/RConn2
  Simulink-PS Converter2/RConn1 -- Controlled Temperature Source2/RConn1
  RY-Z-/LConn1 -- Controlled Temperature Source3/LConn1
  Thermal Reference4/LConn1 -- Controlled Temperature Source3/RConn2
  Simulink-PS Converter3/RConn1 -- Controlled Temperature Source3/RConn1

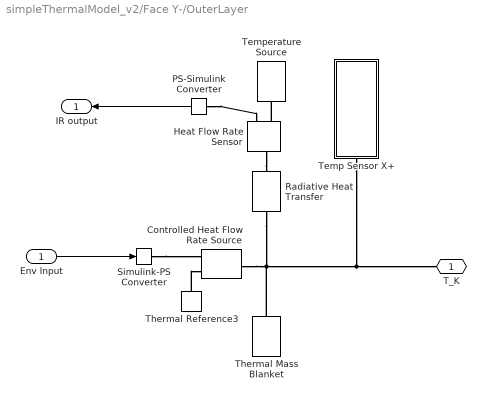
== system simpleThermalModel_v2/Face Y-/OuterLayer ==
  Env Input : Inport
  Controlled Heat Flow Rate Source : fl_lib/Thermal/Thermal Sources/Controlled Heat Flow Rate Source
      settings: SourceProductBaseCode=PW,SS,VE
  Heat Flow Rate Sensor : fl_lib/Thermal/Thermal Sensors/Heat Flow Rate Sensor
      settings: SourceProductBaseCode=PW,SS,VE
  PS-Simulink Converter : nesl_utility/PS-Simulink Converter  PhysicalDomain=network_engine_domain  SubClassName=ps_output  LeftPortType=input  RightPortType=output  PseudoPeriodic=off  Frequencies=[]  VectorFormat=inherit  Unit=inherit  AffineConversion=off
      settings: SourceProductBaseCode=SS,PW,VE
  Radiative Heat Transfer : fl_lib/Thermal/Thermal Elements/Radiative Heat Transfer  area=1 m^2  rad_tr_coeff=1 W/(K^4*m^2)  T_specify=off  T_priority=None  T=0 K  T_nominal_specify=off  T_nominal_unit=K  T_nominal_value=1  Q_specify=off  Q_priority=None  Q=0 W  Q_nominal_specify=off  Q_nominal_unit=W  Q_nominal_value=1
      settings: SourceProductBaseCode=PW,SS,VE  InternalSimscapePortConfiguration="{\"Bottom\":[],\"Left\":[{\"id\":\"A\",\"label\":\"A\",\"type\":\"foundation.thermal.thermal\"}],\"Right\":[{\"id\":\"B\",\"label\":\"B\",\"type\":\"foundation.thermal.thermal\"}],\"Top\":[]}"
  Simulink-PS Converter : nesl_utility/Simulink-PS Converter  PhysicalDomain=network_engine_domain  SubClassName=ps_input  LeftPortType=input  RightPortType=output  PseudoPeriodic=off  Frequencies=[]  NoiseDistribution=none  NoiseParameters=[]  Unit=1  AffineConversion=off  FilteringAndDerivatives=provide  SimscapeFilterOrder=1  InputFilterTimeConstant=0.001  UdotUserProvided=0
      settings: SourceProductBaseCode=SS,PW,VE
  Temp Sensor X+ : Subsystem
  Temperature Source : fl_lib/Thermal/Thermal Sources/Temperature Source  temperature=7 K
      settings: SourceProductBaseCode=PW,SS,VE
  Thermal Mass Blanket : fl_lib/Thermal/Thermal Elements/Thermal Mass  mass=1 kg  sp_heat=1 J/(K*kg)  T_specify=off  T_priority=High  T=300 K  T_nominal_specify=off  T_nominal_unit=K  T_nominal_value=1  Q_specify=off  Q_priority=None  Q=0 W  Q_nominal_specify=off  Q_nominal_unit=W  Q_nominal_value=1
      settings: SourceProductBaseCode=PW,SS,VE
  Thermal Reference3 : fl_lib/Thermal/Thermal Elements/Thermal Reference
      settings: SourceProductBaseCode=PW,SS,VE
  T_K : PMIOPort  Side=Right
  IR output : Outport
  wires:
  Env Input/1 -> Simulink-PS Converter/1
  PS-Simulink Converter/1 -> IR output/1
  connections:
  Controlled Heat Flow Rate Source/LConn1 -- Thermal Mass Blanket/LConn1 -- Radiative Heat Transfer/LConn1 -- Temp Sensor X+/LConn1 -- T_K/RConn1
  Simulink-PS Converter/RConn1 -- Controlled Heat Flow Rate Source/RConn1
  Heat Flow Rate Sensor/LConn1 -- Radiative Heat Transfer/RConn1
  Heat Flow Rate Sensor/RConn2 -- Temperature Source/LConn1
  Thermal Reference3/LConn1 -- Controlled Heat Flow Rate Source/RConn2
  PS-Simulink Converter/LConn1 -- Heat Flow Rate Sensor/RConn1

== system simpleThermalModel_v2/Face Z+/Inner Face Temp ==
  PS-Simulink Converter : nesl_utility/PS-Simulink Converter  PhysicalDomain=network_engine_domain  SubClassName=ps_output  LeftPortType=input  RightPortType=output  PseudoPeriodic=off  Frequencies=[]  VectorFormat=inherit  Unit=inherit  AffineConversion=off
      settings: SourceProductBaseCode=SS,PW,VE
  Temperature Sensor : fl_lib/Thermal/Thermal Sensors/Temperature Sensor
      settings: SourceProductBaseCode=PW,SS,VE
  Thermal Reference1 : fl_lib/Thermal/Thermal Elements/Thermal Reference
      settings: SourceProductBaseCode=PW,SS,VE
  T_K : PMIOPort  Side=Left
  tag scope: InnerFaceTempZplus=global
  wires:
  PS-Simulink Converter/1 -> [InnerFaceTempZplus]
  connections:
  Temperature Sensor/LConn1 -- T_K/RConn1
  Temperature Sensor/RConn2 -- PS-Simulink Converter/LConn1
  Thermal Reference1/LConn1 -- Temperature Sensor/RConn1
